simulink model "phantomx_sim_zero"  (R2025b)
settings: Solver=ode45  StartTime=0.0  StopTime=10.0  MaxStep=1e-3  RelTol=1e-3
InitFcn:
  | % Parametri del filtro
  | num_filters = 18;       % Numero di filtri in parallelo (i tuoi 18 giunti/segnali)
  | tau = 0.05;             % Costante di tempo del filtro in secondi (modificabile)
  | a = 1 / tau;            % Polo del sistema
  | 
  | % 1. Creazione delle Matrici di Stato (State-Space)
  | % Matrice A (Dinamica del sistema): Diagonale con i poli
  | A = -a * eye(num_filters);
  | 
  | % Matrice B (Matrice di ingresso): Diagonale per mappare ogni input al suo stato
  | B = a * eye(num_filters);
  | 
  | % Matrice C (Matrice di uscita): Identità (vogliamo leggere gli stati direttamente)
  | C = eye(num_filters);
  | 
  | % Matrice D (Feedforward): Matrice di zeri (nessun collegamento diretto input-output)
  | D = zeros(num_filters, num_filters);
  | 
  | % 2. Creazione dell'oggetto State-Space in MATLAB
  | sys_filter = ss(A, B, C, D);
  | 
  | % Aggiungiamo i nomi per tenere tutto in ordine (opzionale ma consigliato)
  | sys_filter.InputName = strcat('Action_In_', string(1:num_filters));
  | sys_filter.OutputName = strcat('Filtered_Action_Out_', string(1:num_filters));
  | sys_filter.StateName = strcat('State_', string(1:num_filters));
  | 
  | % Mostra le proprietà del sistema creato
  | disp('Sistema State-Space creato con successo:');
  | sys_filter
values from neighbouring files (symbols this model uses):
  X = rl_actions(idx)    [joint_angles.m]
  Y = -Y    [joint_angles.m]
  Z = rl_actions(idx+2)    [joint_angles.m]
libraries: sm_lib x237, nesl_utility x40, rllib x1
(part 5 of 5)

== system phantomx_sim_zero/tibia_rr ==
  Inertia : sm_lib/Body Elements/Inertia  InertiaType=Custom  Mass=0.024357719  MassUnits=kg  CenterOfMass=[0, 0, 0]  CenterOfMassUnits=m  MomentsOfInertia=[0.0051411124, 0.0081915737, 0.0011379812]  MomentsOfInertiaUnits=kg*m^2  ProductsOfInertia=[-1.9223094e-05, -2.4729049e-05, -0.0005753025500000001]  ProductsOfInertiaUnits=kg*m^2  GraphicType=None  MarkerShape=Inertia  MarkerSize=20  GraphicVisPropType=SimpleVisualProperties  GraphicDiffuseColor=[0.5 0.5 0.5]  GraphicOpacity=1  GraphicSpecularColor=[0.5 0.5 0.5 1.0]  GraphicAmbientColor=[0.15 0.15 0.15 1.0]  GraphicEmissiveColor=[0.0 0.0 0.0 1.0]  GraphicShininess=75
  InertiaOriginTransform : sm_lib/Frames and Transforms/Rigid Transform  RotationMethod=RotationSequence  FollAlignAxisA=+X  BaseAlignAxisA=+Y  FollAlignAxisB=+Y  BaseAlignAxisB=+Z  RotationStandardAxis=+Z  RotationAngle=0  RotationAngleUnits=deg  RotationArbitraryAxis=[0 0 1]  RotationSequenceAxes=BaseAxes  RotationSequence=XYZ  RotationSequenceAngles=[0, 0, 0]  RotationSequenceAnglesUnits=rad  RotationMatrix=[1 0 0;0 1 0;0 0 1]  Quaternion=[1 0 0 0]  TranslationMethod=Cartesian  TranslationCartesianOffset=[0, 0, 0]  TranslationCartesianOffsetUnits=m  TranslationStandardAxis=+Z  TranslationStandardOffset=0  TranslationStandardOffsetUnits=m  TranslationROffset=0  TranslationROffsetUnits=m  TranslationThetaOffset=0  TranslationThetaOffsetUnits=deg  TranslationZOffset=0  TranslationZOffsetUnits=m
  ReferenceFrame : sm_lib/Frames and Transforms/Reference Frame
  Visual : sm_lib/Body Elements/File Solid  ExtGeomFileName=meshes/tibia_l.STL  UnitType=Custom  ExtGeomFileUnits=m  StepReaderType=HEX  ExportConvexHullGeometry=off  InertiaType=Custom  BasedOnType=DensityFromFile  Density=1000  DensityUnits=kg/m^3  Mass=0  MassUnits=kg  CenterOfMass=[0, 0, 0]  CenterOfMassUnits=m  MomentsOfInertia=[0, 0, 0]  MomentsOfInertiaUnits=kg*m^2  ProductsOfInertia=[0, 0, 0]  ProductsOfInertiaUnits=kg*m^2  GraphicType=FromGeometry  MarkerShape=Sphere  MarkerSize=10  GraphicVisPropType=SimpleVisualProperties  GraphicDiffuseColor=[0.2, 0.2, 0.2]  GraphicOpacity=1  GraphicSpecularColor=[0.5 0.5 0.5 1.0]  GraphicAmbientColor=[0.15 0.15 0.15 1.0]  GraphicEmissiveColor=[0.0 0.0 0.0 1.0]  GraphicShininess=75  DoExposeReferenceFrame=on  SerializedFrames=<Frames/>
  VisualOriginTransform : sm_lib/Frames and Transforms/Rigid Transform  RotationMethod=RotationSequence  FollAlignAxisA=+X  BaseAlignAxisA=+Y  FollAlignAxisB=+Y  BaseAlignAxisB=+Z  RotationStandardAxis=+Z  RotationAngle=0  RotationAngleUnits=deg  RotationArbitraryAxis=[0 0 1]  RotationSequenceAxes=BaseAxes  RotationSequence=XYZ  RotationSequenceAngles=[0, 0, 0]  RotationSequenceAnglesUnits=rad  RotationMatrix=[1 0 0;0 1 0;0 0 1]  Quaternion=[1 0 0 0]  TranslationMethod=Cartesian  TranslationCartesianOffset=[0, 0, 0]  TranslationCartesianOffsetUnits=m  TranslationStandardAxis=+Z  TranslationStandardOffset=0  TranslationStandardOffsetUnits=m  TranslationROffset=0  TranslationROffsetUnits=m  TranslationThetaOffset=0  TranslationThetaOffsetUnits=deg  TranslationZOffset=0  TranslationZOffsetUnits=m
  j_tibia_rr_AxisInvTransform : sm_lib/Frames and Transforms/Rigid Transform  RotationMethod=ArbitraryAxis  FollAlignAxisA=+X  BaseAlignAxisA=+Y  FollAlignAxisB=+Y  BaseAlignAxisB=+Z  RotationStandardAxis=+Z  RotationAngle=1.570796326794897  RotationAngleUnits=rad  RotationArbitraryAxis=[-0, 1, 0]  RotationSequenceAxes=FollowerAxes  RotationSequence=XYX  RotationSequenceAngles=[0 0 0]  RotationSequenceAnglesUnits=deg  RotationMatrix=[1 0 0;0 1 0;0 0 1]  Quaternion=[1 0 0 0]  TranslationMethod=Cartesian  TranslationCartesianOffset=[0, 0, 0]  TranslationCartesianOffsetUnits=m  TranslationStandardAxis=+Z  TranslationStandardOffset=0  TranslationStandardOffsetUnits=m  TranslationROffset=0  TranslationROffsetUnits=m  TranslationThetaOffset=0  TranslationThetaOffsetUnits=deg  TranslationZOffset=0  TranslationZOffsetUnits=m
  F : PMIOPort  Side=Left
  connections:
  Inertia/RConn1 -- InertiaOriginTransform/RConn1
  ReferenceFrame/RConn1 -- InertiaOriginTransform/LConn1 -- VisualOriginTransform/LConn1 -- j_tibia_rr_AxisInvTransform/LConn1
  Visual/RConn1 -- VisualOriginTransform/RConn1
  j_tibia_rr_AxisInvTransform/RConn1 -- F/RConn1

== matlab function phantomx_sim_zero/MR ==
  data: x input; theta output; y input; z input; phi output; psi output; side input; alpha input
function [theta, phi, psi] = inv_kyn(x, y, z, side, alpha)
    %#codegen
    % x: Comando spostamento AVANTI (+X = avanti)
    % y: Comando spostamento LATERALE (+Y = sinistra)
    % z: Comando ALTEZZA (+Z = basso)
    % side: +1 per zampe Sinistre, -1 per zampe Destre
    % alpha: Angolo di montaggio rispetto all'asse X del corpo (in radianti)

    % Offset di Posizione a riposo (Postura)
    r_offset = 0.12; % 12 cm di estensione radiale base

    % Parametri geometrici dei link (in metri)
    lc = 0.054;
    lf = 0.0661;
    lt = 0.12;

    % 1. Trasformazione Matriziale dal Paper: R_z(-alpha) * P_body
    x_loc = r_offset + x * cos(alpha) + y * sin(alpha);
    y_loc = (-x * sin(alpha) + y * cos(alpha)) * side;
    z_loc = z;

    % 2. Cinematica Inversa Locale
    trueX = sqrt(x_loc*x_loc + y_loc*y_loc) - lc;
    im = sqrt(trueX*trueX + z_loc*z_loc);

    % Coxa (theta)
    theta = -atan2(y_loc, x_loc)*side;

    % Femore (phi)
    term_phi = (lf*lf + im*im - lt*lt) / (2 * im * lf);
    term_phi = max(-1.0, min(1.0, term_phi));
    phi = (pi/2) - atan2(trueX, z_loc) - acos(term_phi);

    % Tibia (psi)
    term_psi = (lf*lf - im*im + lt*lt) / (2 * lt * lf);
    term_psi = max(-1.0, min(1.0, term_psi));
    psi = pi - acos(term_psi);

    % Inversione segno giunto Simscape
    psi = -psi;
end

== matlab function phantomx_sim_zero/RR ==
  data: x input; theta output; y input; z input; phi output; psi output; side input; alpha input
function [theta, phi, psi] = inv_kyn(x, y, z, side, alpha)
    %#codegen
    % x: Comando spostamento AVANTI (+X = avanti)
    % y: Comando spostamento LATERALE (+Y = sinistra)
    % z: Comando ALTEZZA (+Z = basso)
    % side: +1 per zampe Sinistre, -1 per zampe Destre
    % alpha: Angolo di montaggio rispetto all'asse X del corpo (in radianti)

    % Offset di Posizione a riposo (Postura)
    r_offset = 0.12; % 12 cm di estensione radiale base

    % Parametri geometrici dei link (in metri)
    lc = 0.054;
    lf = 0.0661;
    lt = 0.12;

    % 1. Trasformazione Matriziale dal Paper: R_z(-alpha) * P_body
    x_loc = r_offset + x * cos(alpha) + y * sin(alpha);
    y_loc = (-x * sin(alpha) + y * cos(alpha)) * side;
    z_loc = z;

    % 2. Cinematica Inversa Locale
    trueX = sqrt(x_loc*x_loc + y_loc*y_loc) - lc;
    im = sqrt(trueX*trueX + z_loc*z_loc);

    % Coxa (theta)
    theta = -atan2(y_loc, x_loc)*side;

    % Femore (phi)
    term_phi = (lf*lf + im*im - lt*lt) / (2 * im * lf);
    term_phi = max(-1.0, min(1.0, term_phi));
    phi = (pi/2) - atan2(trueX, z_loc) - acos(term_phi);

    % Tibia (psi)
    term_psi = (lf*lf - im*im + lt*lt) / (2 * lt * lf);
    term_psi = max(-1.0, min(1.0, term_psi));
    psi = pi - acos(term_psi);

    % Inversione segno giunto Simscape
    psi = -psi;
end

== matlab function phantomx_sim_zero/FR ==
  data: x input; theta output; y input; z input; phi output; psi output; side input; alpha input
function [theta, phi, psi] = inv_kyn(x, y, z, side, alpha)
    %#codegen
    % x: Comando spostamento AVANTI (+X = avanti)
    % y: Comando spostamento LATERALE (+Y = sinistra)
    % z: Comando ALTEZZA (+Z = basso)
    % side: +1 per zampe Sinistre, -1 per zampe Destre
    % alpha: Angolo di montaggio rispetto all'asse X del corpo (in radianti)

    % Offset di Posizione a riposo (Postura)
    r_offset = 0.12; % 12 cm di estensione radiale base

    % Parametri geometrici dei link (in metri)
    lc = 0.054;
    lf = 0.0661;
    lt = 0.12;

    % 1. Trasformazione Matriziale dal Paper: R_z(-alpha) * P_body
    x_loc = r_offset + x * cos(alpha) + y * sin(alpha);
    y_loc = (-x * sin(alpha) + y * cos(alpha)) * side;
    z_loc = z;

    % 2. Cinematica Inversa Locale
    trueX = sqrt(x_loc*x_loc + y_loc*y_loc) - lc;
    im = sqrt(trueX*trueX + z_loc*z_loc);

    % Coxa (theta)
    theta = -atan2(y_loc, x_loc)*side;

    % Femore (phi)
    term_phi = (lf*lf + im*im - lt*lt) / (2 * im * lf);
    term_phi = max(-1.0, min(1.0, term_phi));
    phi = (pi/2) - atan2(trueX, z_loc) - acos(term_phi);

    % Tibia (psi)
    term_psi = (lf*lf - im*im + lt*lt) / (2 * lt * lf);
    term_psi = max(-1.0, min(1.0, term_psi));
    psi = pi - acos(term_psi);

    % Inversione segno giunto Simscape
    psi = -psi;
end

== matlab function phantomx_sim_zero/RL ==
  data: x input; theta output; y input; z input; phi output; psi output; side input; alpha input
function [theta, phi, psi] = inv_kyn(x, y, z, side, alpha)
    %#codegen
    % x: Comando spostamento AVANTI (+X = avanti)
    % y: Comando spostamento LATERALE (+Y = sinistra)
    % z: Comando ALTEZZA (+Z = basso)
    % side: +1 per zampe Sinistre, -1 per zampe Destre
    % alpha: Angolo di montaggio rispetto all'asse X del corpo (in radianti)

    % Offset di Posizione a riposo (Postura)
    r_offset = 0.12; % 12 cm di estensione radiale base
    
    % Parametri geometrici dei link (in metri)
    lc = 0.054;
    lf = 0.0661;
    lt = 0.12;

    % 1. Trasformazione Matriziale dal Paper: R_z(-alpha) * P_body
    x_loc = r_offset + x * cos(alpha) + y * sin(alpha);
    y_loc = (-x * sin(alpha) + y * cos(alpha)) * side;
    z_loc = z;

    % 2. Cinematica Inversa Locale
    trueX = sqrt(x_loc*x_loc + y_loc*y_loc) - lc;
    im = sqrt(trueX*trueX + z_loc*z_loc);

    % Coxa (theta)
    theta = atan2(y_loc, x_loc)*side;

    % Femore (phi)
    term_phi = (lf*lf + im*im - lt*lt) / (2 * im * lf);
    term_phi = max(-1.0, min(1.0, term_phi));
    phi = (pi/2) - atan2(trueX, z_loc) - acos(term_phi);

    % Tibia (psi)
    term_psi = (lf*lf - im*im + lt*lt) / (2 * lt * lf);
    term_psi = max(-1.0, min(1.0, term_psi));
    psi = pi - acos(term_psi);

    % Inversione segno giunto Simscape
    psi = -psi;
end

== matlab function phantomx_sim_zero/ML ==
  data: x input; theta output; y input; z input; phi output; psi output; side input; alpha input
function [theta, phi, psi] = inv_kyn(x, y, z, side, alpha)
    %#codegen
    % x: Comando spostamento AVANTI (+X = avanti)
    % y: Comando spostamento LATERALE (+Y = sinistra)
    % z: Comando ALTEZZA (+Z = basso)
    % side: +1 per zampe Sinistre, -1 per zampe Destre
    % alpha: Angolo di montaggio rispetto all'asse X del corpo (in radianti)

    % Offset di Posizione a riposo (Postura)
    r_offset = 0.12; % 12 cm di estensione radiale base

    % Parametri geometrici dei link (in metri)
    lc = 0.054;
    lf = 0.0661;
    lt = 0.12;

    % 1. Trasformazione Matriziale dal Paper: R_z(-alpha) * P_body
    x_loc = r_offset + x * cos(alpha) + y * sin(alpha);
    y_loc = (-x * sin(alpha) + y * cos(alpha)) * side;
    z_loc = z;

    % 2. Cinematica Inversa Locale
    trueX = sqrt(x_loc*x_loc + y_loc*y_loc) - lc;
    im = sqrt(trueX*trueX + z_loc*z_loc);

    % Coxa (theta)
    theta = atan2(y_loc, x_loc)*side;

    % Femore (phi)
    term_phi = (lf*lf + im*im - lt*lt) / (2 * im * lf);
    term_phi = max(-1.0, min(1.0, term_phi));
    phi = (pi/2) - atan2(trueX, z_loc) - acos(term_phi);

    % Tibia (psi)
    term_psi = (lf*lf - im*im + lt*lt) / (2 * lt * lf);
    term_psi = max(-1.0, min(1.0, term_psi));
    psi = pi - acos(term_psi);

    % Inversione segno giunto Simscape
    psi = -psi;
end

== matlab function phantomx_sim_zero/FL ==
  data: x input; theta output; y input; z input; phi output; psi output; side input; alpha input
function [theta, phi, psi] = inv_kyn(x, y, z, side, alpha)
    %#codegen
    % x: Comando spostamento AVANTI (+X = avanti)
    % y: Comando spostamento LATERALE (+Y = sinistra)
    % z: Comando ALTEZZA (+Z = basso)
    % side: +1 per zampe Sinistre, -1 per zampe Destre
    % alpha: Angolo di montaggio rispetto all'asse X del corpo (in radianti)

    % Offset di Posizione a riposo (Postura)
    r_offset = 0.12; % 12 cm di estensione radiale base

    % Parametri geometrici dei link (in metri)
    lc = 0.054;
    lf = 0.0661;
    lt = 0.12;

    % 1. Trasformazione Matriziale dal Paper: R_z(-alpha) * P_body
    x_loc = r_offset + x * cos(alpha) + y * sin(alpha);
    y_loc = (-x * sin(alpha) + y * cos(alpha)) * side;
    z_loc = z;

    % 2. Cinematica Inversa Locale
    trueX = sqrt(x_loc*x_loc + y_loc*y_loc) - lc;
    im = sqrt(trueX*trueX + z_loc*z_loc);

    % Coxa (theta)
    theta = atan2(y_loc, x_loc)*side;

    % Femore (phi)
    term_phi = (lf*lf + im*im - lt*lt) / (2 * im * lf);
    term_phi = max(-1.0, min(1.0, term_phi));
    phi = (pi/2) - atan2(trueX, z_loc) - acos(term_phi);

    % Tibia (psi)
    term_psi = (lf*lf - im*im + lt*lt) / (2 * lt * lf);
    term_psi = max(-1.0, min(1.0, term_psi));
    psi = pi - acos(term_psi);

    % Inversione segno giunto Simscape
    psi = -psi;
end
